simulink model "spec_Resident_Task44"  (R2016b)
settings: Solver=ode45  StartTime=0  StopTime=365*24*3600  RelTol=1e-3  EnableMultiTasking=on
InitFcn:
  | load('DE_TRY2010_04_averageYear')
undefined symbols (not defined in the file): path_carnot
libraries: carnot x2
settings Model: Creator=drhf  LastModifiedBy=drhf
settings DataIOCC: SaveFormat=Array  SignalLoggingSaveFormat=ModelDataLogs
settings OptimizationCC: ExpressionDepthLimit=2147483647  LifeSpan=inf
settings DebuggingCC: UnderspecifiedInitializationDetection=Classic  MergeDetectMultiDrivingBlocksExec=none  SolverPrmCheckMsg=warning  FcnCallInpInsideContextMsg=warning  StateNameClashWarn=warning  SFUnexpectedBacktrackingDiag=warning  SFNoUnconditionalDefaultTransitionDiag=warning  SFExecutionAtInitializationDiag=none
settings HardwareCC: ProdBitPerPointer=32  ProdBitPerSizeT=32  ProdBitPerPtrDiffT=32  ProdLargestAtomicFloat=None  ProdIntDivRoundTo=Undefined  ProdEndianess=Unspecified  ProdWordSize=32  ProdHWDeviceType=32-bit Generic
settings ModelReferenceCC: PropagateSignalLabelsOutOfModel=off
settings GRTTargetCC: TargetLangStandard=C89/C90 (ANSI)  GeneratePreprocessorConditionals=Disable all  CombineOutputUpdateFcns=off  GRTInterface=on
settings ConfigComp: CovMetricSettings=dw  CovHtmlReporting=on  CovSaveCumulativeToWorkspaceVar=on  CovSaveSingleToWorkspaceVar=on  CovExternalEMLEnable=off

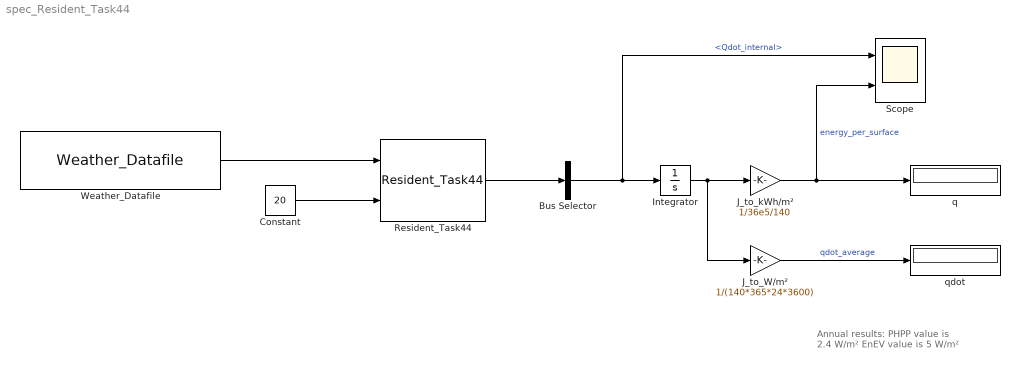
== system spec_Resident_Task44 ==
  note: Annual results:
      | PHPP value is 2.4 W/m²
      | EnEV value is 5 W/m²
  Bus Selector : BusSelector  OutputSignals=Qdot_internal
  Constant : Constant  Value=20
  Integrator : Integrator
  J_to_W/m² : Gain  Gain=1/(140*365*24*3600)
  J_to_kWh/m² : Gain  Gain=1/36e5/140
  Resident_Task44 : carnot/Load/Houses/Resident_Task44  period=24*3600  rep_seq_te=[0 1 6 7 8 9 11 12 13 18 19 20 22 23]*3600  rep_seq_de=[1 5 1 1 1 2 1 1 4 2 1 2 1 1]*3600  rep_seq_ye=[105 55 392.5 457.5 420 55 250 55 120 170 615 420 442.5 355]  rep_seq_to=[0 6 7 8 9 11 12 13 14 15 17 18 20 21 22]*3600  rep_seq_do=[6 1 1 1 2 1 1 1 1 2 1 2 1 1 2]*3600  rep_seq_yo=[4 2 3 2 0 1 3 2 1 0 1 2 4 3 4]*60  Topen=24  Tclose=23  TrAboveTa=2  TaTooCold=12  timeFIR=24  TaIni=12  starttime=8  stoptime=22  TroomShadeOn=23.8  TroomShadeOff=22.8  SolarShadeOn=300  SolarShadeOff=200  max_shade=1  CalcAirComp=on  mdotCO2=0  mdotH2O=0  mdotVOC=0
  Scope : Scope  NumInputPorts=2
  Weather_Datafile : carnot/Weather/Weather_Datafile  PathName=path_carnot('data')  FileName='DE_TRY2010_04_averageYear.mat'  UserParam=off  VariableName=DE_TRY2010_04_averageYear  SampleTime=3600
  q : Display
  qdot : Display
  wires:
  Integrator/1 -> J_to_W/m²/1, J_to_kWh/m²/1
  J_to_kWh/m²/1 -> Scope/2, q/1  "energy_per_surface"
  Weather_Datafile/1 -> Resident_Task44/1
  Resident_Task44/1 -> Bus Selector/1
  Constant/1 -> Resident_Task44/2
  Bus Selector/1 -> Integrator/1, Scope/1  "<Qdot_internal>"
  J_to_W/m²/1 -> qdot/1  "qdot_average"
